simulink model "UDP_INTEGRATION_TEST_01"  (Simulink 8.1)
settings: Solver=ode4  StartTime=0.0  StopTime=inf  FixedStep=Ts  MaxStep=1e-3  RelTol=1e-3
PostLoadFcn:
  | INTEGRATION_TEST_01_init;
InitFcn:
  | INTEGRATION_TEST_01_init;
values from neighbouring files (symbols this model uses):
  Ts = 100E-6    (= 0.0001)    [INTEGRATION_TEST_01_init.m]
undefined symbols (not defined in the file or in its folder): cable_spec, fdesignblkfcn, gcbh, Left, relay_par, type, V
libraries: powerlib_extras x14, rtio_opalrt_common x13, rtlab x8, cables_lib x6, breaker_lib x4, simulink_extras x4, simulink x4, Load_lib x3, rtio_generic_modbus x3, powerlib x2, ssn_lib x2, transformer_lib x2
(part 2 of 2)

== system UDP_INTEGRATION_TEST_01/SS_Relays_and_Woodward/HWCtrl/SEL751_DigitalAnalog_IO_OpBlocks ==
  note: This connector also services Genset #2 and  is
      | shared with Genset #1.  Use RJ45 connectors to
      |  intercept Genset #2 I/O (not used in this Device
      | Integration Test) and use for SEL-751
  note: Remove existing connections to Slot 3 I/O, if any
      | ans replace with connections shown below, or use
      | corresponding RJ45 connectors.  (Existing I/O, if any not
      |  used for this Device Integration Test)
  note: When the system uses the simulated
      | Secondary Controller the digital I/O
      | should be disabled.
  note: Copyright (c) 2016 Massachusetts Institute of Technology
      | Permission is hereby granted, free of charge, to any person obtaining a copy of this software and associated documentation files (the "Software"), to deal
      | in the Software without restriction, including without limitation the rights to use, copy, modify, merge, publish, distribute, sublicense, and/or sell copies of the
      | Software, and to permit persons to whom the Software is furnished to do so, subject to the following conditions:
      |
      | THE SOFTWARE IS PROVIDED "AS IS", WITHOUT WARRANTY OF ANY KIND, EXPRESS OR IMPLIED, INCLUDING BUT NOT LIMITED TO THE
      | WARRANTIES OF MERCHANTABILITY, FITNESS FOR A PARTICULAR PURPOSE AND NONINFRINGEMENT. IN NO EVENT SHALL THE AUTHORS
      | OR COPYRIGHT HOLDERS BE LIABLE FOR ANY CLAIM, DAMAGES OR OTHER LIABILITY, WHETHER IN AN ACTION OF CONTRACT, TORT OR
      | OTHERWISE, ARISING FROM, OUT OF OR IN CONNECTION WITH THE SOFTWARE OR THE USE OR OTHER DEALINGS IN THE SOFTWARE
  SEL751-01_ScaledSignals : Inport
  AnalogOut2 to SEL-751 : rtio_opalrt_common/AnalogOut  CtrlName='OpCtrl'  portNb=4  FcnNos=Slot 2 Module A Subsection 2  size=16  maxcount=8  count=8  numchan=8  israngeinput=off  voltagerange=[ -5 ... 5 ]  slot=1  side=0  mismatch=0  slotside=Slot_2_Module_A
      settings: AttributesFormatString=%<CtrlName>
  Bus Creator4 : BusCreator  Inputs=2
  Bus Selector4 : BusSelector  OutputSignals=To DigitalOut_to_SEL-751,To AnalogOut_to_SEL-751
  Data Type Conversion{,1..3} (4 alike) : DataTypeConversion
  Demux6 : Demux  Outputs=8
  DigitalIn from SEL-751 : rtio_opalrt_common/DigitalIn  CtrlName='OpCtrl'  portNb=6  FcnNos=Slot 3 Module A Subsection 2  size=1  maxcount=8  count=8  sampleTime=Ts  numchan=8
      settings: AttributesFormatString=%<CtrlName>
  DigitalOut to SEL-751 : rtio_opalrt_common/DigitalOut  CtrlName='OpCtrl'  portNb=6  FcnNos=Slot 3 Module B Subsection 2  size=1  maxcount=8  count=8  numchan=8
      settings: AttributesFormatString=%<CtrlName>
  S-R Flip-Flop : simulink_extras/Flip Flops/S-R Flip-Flop  initial_condition=1
  Terminator : Terminator
  Terminator1 : Terminator
  Terminator2 : Terminator
  SEL751-01_LogicTrip : Outport
  wires:
  DigitalOut to SEL-751/1 -> Terminator1/1
  AnalogOut2 to SEL-751/1 -> Terminator/1
  Demux6/2 -> Data Type Conversion1/1  "OUT102 Brkr reset"
  Demux6/1 -> Data Type Conversion/1  "OUT103 Brkr trip"
  Data Type Conversion3/1 -> Bus Creator4/2  "Logic_reset"
  Data Type Conversion/1 -> S-R Flip-Flop/1
  Bus Selector4/2 -> AnalogOut2 to SEL-751/1  "<To AnalogOut_to_SEL-751>"
  Bus Selector4/1 -> DigitalOut to SEL-751/1  "<To DigitalOut_to_SEL-751>"
  DigitalIn from SEL-751/2 -> Terminator2/1
  SEL751-01_ScaledSignals/1 -> Bus Selector4/1
  DigitalIn from SEL-751/1 -> Demux6/1
  Data Type Conversion1/1 -> S-R Flip-Flop/2
  Data Type Conversion2/1 -> Bus Creator4/1  "Logic_trip"
  Bus Creator4/1 -> SEL751-01_LogicTrip/1
  S-R Flip-Flop/1 -> Data Type Conversion2/1  "Logic_trip"
  S-R Flip-Flop/2 -> Data Type Conversion3/1  "Logic_reset"

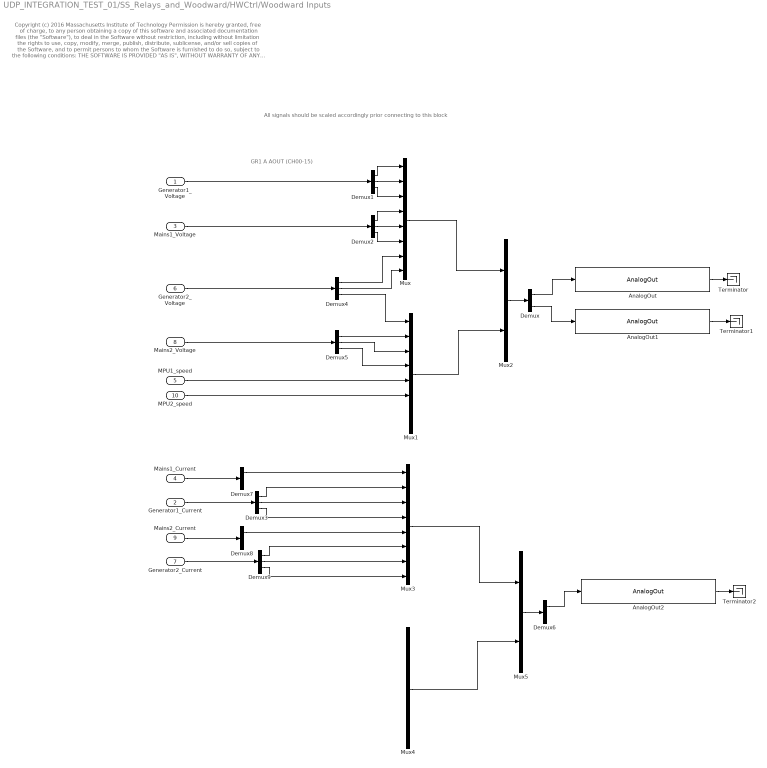
== system UDP_INTEGRATION_TEST_01/SS_Relays_and_Woodward/HWCtrl/Woodward Inputs ==
  note: All signals should be scaled accordingly prior connecting to this block
  note: GR1 A AOUT (CH00-15)
  note: Copyright (c) 2016 Massachusetts Institute of Technology
      | Permission is hereby granted, free of charge, to any person obtaining a copy of this software and associated documentation files (the "Software"), to deal
      | in the Software without restriction, including without limitation the rights to use, copy, modify, merge, publish, distribute, sublicense, and/or sell copies of the
      | Software, and to permit persons to whom the Software is furnished to do so, subject to the following conditions:
      |
      | THE SOFTWARE IS PROVIDED "AS IS", WITHOUT WARRANTY OF ANY KIND, EXPRESS OR IMPLIED, INCLUDING BUT NOT LIMITED TO THE
      | WARRANTIES OF MERCHANTABILITY, FITNESS FOR A PARTICULAR PURPOSE AND NONINFRINGEMENT. IN NO EVENT SHALL THE AUTHORS
      | OR COPYRIGHT HOLDERS BE LIABLE FOR ANY CLAIM, DAMAGES OR OTHER LIABILITY, WHETHER IN AN ACTION OF CONTRACT, TORT OR
      | OTHERWISE, ARISING FROM, OUT OF OR IN CONNECTION WITH THE SOFTWARE OR THE USE OR OTHER DEALINGS IN THE SOFTWARE
  Generator1_Voltage : Inport
  Generator1_Current : Inport  Port=2
  Mains1_Voltage : Inport  Port=3
  Mains1_Current : Inport  Port=4
  MPU1_speed : Inport  Port=5
  Generator2_Voltage : Inport  Port=6
  Generator2_Current : Inport  Port=7
  Mains2_Voltage : Inport  Port=8
  Mains2_Current : Inport  Port=9
  MPU2_speed : Inport  Port=10
  AnalogOut : rtio_opalrt_common/AnalogOut  CtrlName='OpCtrl'  portNb=1  FcnNos=Slot 1 Module A Subsection 1  size=16  maxcount=8  count=8  numchan=8  israngeinput=off  voltagerange=[-16 ... 16]  slot=0  side=0  mismatch=0  slotside=Slot_1_Module_A
      settings: AttributesFormatString=%<CtrlName>
  AnalogOut1 : rtio_opalrt_common/AnalogOut  CtrlName='OpCtrl'  portNb=2  FcnNos=Slot 1 Module A Subsection 2  size=16  maxcount=8  count=8  numchan=8  israngeinput=off  voltagerange=[-16 ... 16]  slot=0  side=0  mismatch=0  slotside=Slot_1_Module_A
      settings: AttributesFormatString=%<CtrlName>
  AnalogOut2 : rtio_opalrt_common/AnalogOut  CtrlName='OpCtrl'  portNb=3  FcnNos=Slot 2 Module A Subsection 1  size=16  maxcount=8  count=8  numchan=8  israngeinput=off  voltagerange=[-16 ... 16]  slot=1  side=0  mismatch=0  slotside=Slot_2_Module_A
      settings: AttributesFormatString=%<CtrlName>
  Demux : Demux  Outputs=2
  Demux{1..5,7..9} (8 alike) : Demux  Outputs=3
  Demux6 : Demux  Outputs=2
  Mux{,1,3..4} (4 alike) : Mux  Inputs=8
  Mux2 : Mux  Inputs=2
  Mux5 : Mux  Inputs=2
  Terminator : Terminator
  Terminator1 : Terminator
  Terminator2 : Terminator
  wires:
  Demux9/3 -> Mux3/8
  Demux9/2 -> Mux3/7
  Demux9/1 -> Mux3/6
  Generator2_Current/1 -> Demux9/1
  Demux8/1 -> Mux3/5
  Mains2_Current/1 -> Demux8/1
  MPU2_speed/1 -> Mux1/6
  Generator2_Voltage/1 -> Demux4/1
  Mains2_Voltage/1 -> Demux5/1
  Demux7/1 -> Mux3/1
  Mains1_Current/1 -> Demux7/1
  Demux3/3 -> Mux3/4
  Demux3/2 -> Mux3/3
  Demux3/1 -> Mux3/2
  Generator1_Current/1 -> Demux3/1
  AnalogOut2/1 -> Terminator2/1
  Demux6/1 -> AnalogOut2/1
  Mux3/1 -> Mux5/1
  Mux4/1 -> Mux5/2
  Mux5/1 -> Demux6/1
  Demux5/3 -> Mux1/4
  Demux5/2 -> Mux1/3
  Demux5/1 -> Mux1/2
  Demux4/3 -> Mux1/1
  Demux4/2 -> Mux/8
  Demux4/1 -> Mux/7
  MPU1_speed/1 -> Mux1/5
  Demux2/3 -> Mux/6
  Demux2/2 -> Mux/5
  Demux2/1 -> Mux/4
  Demux1/3 -> Mux/3
  Demux1/2 -> Mux/2
  Demux1/1 -> Mux/1
  AnalogOut/1 -> Terminator/1
  AnalogOut1/1 -> Terminator1/1
  Demux/1 -> AnalogOut/1
  Demux/2 -> AnalogOut1/1
  Mux/1 -> Mux2/1
  Mux1/1 -> Mux2/2
  Mux2/1 -> Demux/1
  Generator1_Voltage/1 -> Demux1/1
  Mains1_Voltage/1 -> Demux2/1

== system UDP_INTEGRATION_TEST_01/SS_Relays_and_Woodward/HWCtrl/Woodward Outputs - NGCHP - Gen1 ==
  note: Copyright (c) 2016 Massachusetts Institute of Technology
      | Permission is hereby granted, free of charge, to any person obtaining a copy of this software and associated documentation files (the "Software"), to deal
      | in the Software without restriction, including without limitation the rights to use, copy, modify, merge, publish, distribute, sublicense, and/or sell copies of the
      | Software, and to permit persons to whom the Software is furnished to do so, subject to the following conditions:
      |
      | THE SOFTWARE IS PROVIDED "AS IS", WITHOUT WARRANTY OF ANY KIND, EXPRESS OR IMPLIED, INCLUDING BUT NOT LIMITED TO THE
      | WARRANTIES OF MERCHANTABILITY, FITNESS FOR A PARTICULAR PURPOSE AND NONINFRINGEMENT. IN NO EVENT SHALL THE AUTHORS
      | OR COPYRIGHT HOLDERS BE LIABLE FOR ANY CLAIM, DAMAGES OR OTHER LIABILITY, WHETHER IN AN ACTION OF CONTRACT, TORT OR
      | OTHERWISE, ARISING FROM, OUT OF OR IN CONNECTION WITH THE SOFTWARE OR THE USE OR OTHER DEALINGS IN THE SOFTWARE
  Gen1 MCB Status : Inport
  WoodwardBias : Inport  Port=2
  Bus Creator1 : BusCreator  Inputs=1
  DIO - Gr3 : Subsystem
  DIO - Woodward : Subsystem
  DOUT type config : Subsystem
  Woodward Primary Inputs - Gen1 : Subsystem
  Digital Inputs : Outport
  Gen1 Gov and AVR : Outport  Port=2
  Gen1 Fuel Enable : Outport  Port=3
  Gen1 GCB : Outport  Port=4
  Gen1 MCB : Outport  Port=5
  wires:
  Gen1 MCB Status/1 -> DIO - Woodward/2(Gen1 MCB Status)
  DIO - Woodward/1(Gen1 Fuel Enable) -> Gen1 Fuel Enable/1
  DIO - Woodward/3(Gen1 MCB) -> Gen1 MCB/1
  DIO - Woodward/2(Gen1 GCB) -> Gen1 GCB/1
  WoodwardBias/1 -> Woodward Primary Inputs - Gen1/1(WoodwardBias)
  Woodward Primary Inputs - Gen1/1(Gen1 Gov and AVR) -> Gen1 Gov and AVR/1
  Bus Creator1/1 -> Digital Inputs/1
  DIO - Gr3/1(DIn) -> Bus Creator1/1, DIO - Woodward/1(Din_Wood)  "DIN"
  DIO - Woodward/4(DIn1) -> DIO - Gr3/1(Dout)

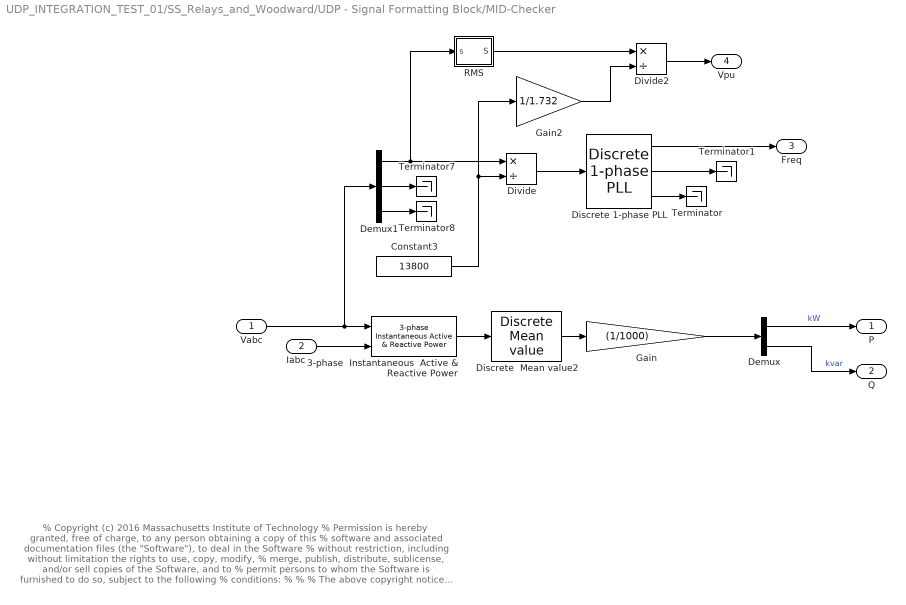
== system UDP_INTEGRATION_TEST_01/SS_Relays_and_Woodward/UDP - Signal Formatting Block/MID-Checker ==
  note: % Copyright (c) 2016 Massachusetts Institute of Technology
      | % Permission is hereby granted, free of charge, to any person obtaining a copy of this
      | % software and associated documentation files (the "Software"), to deal in the Software
      | % without restriction, including without limitation the rights to use, copy, modify,
      | % merge, publish, distribute, sublicense, and/or sell copies of the Software, and to
      | % permit persons to whom the Software is furnished to do so, subject to the following
      | % conditions:
      | %
      | %
      | % The above copyright notice and this permission notice shall be included in
      | % all copies or substantial portions of the Software.
      | %
      | % THE SOFTWARE IS PROVIDED "AS IS", WITHOUT WARRANTY OF ANY KIND, EXPRESS OR IMPLIED,
      | % INCLUDING BUT NOT LIMITED TO THE WARRANTIES OF MERCHANTABILITY, FITNESS FOR A
      | % PARTICULAR PURPOSE AND NONINFRINGEMENT. IN NO EVENT SHALL THE AUTHORS OR COPYRIGHT
      | % HOLDERS BE LIABLE FOR ANY CLAIM, DAMAGES OR OTHER LIABILITY, WHETHER IN AN ACTION
      | % OF CONTRACT, TORT OR OTHERWISE, ARISING FROM, OUT OF OR IN CONNECTION WITH THE
      | % SOFTWARE OR THE USE OR OTHER DEALINGS IN THE SOFTWARE.
      | %
      | %
      | %%
  Vabc : Inport
  Iabc : Inport  Port=2
  3-phase  Instantaneous  Active & Reactive Power : powerlib_extras/Measurements/3-phase  Instantaneous  Active & Reactive Power
  Constant3 : Constant  Value=13800
  Demux : Demux  Outputs=2
  Demux1 : Demux  Outputs=3
  Discrete 1-phase PLL : powerlib_extras/Discrete  Control Blocks/Discrete 1-phase PLL  Fmin=45  Par_Init=[0 60]  ParK=[ 180 3200 1]  Ts=Ts  AGC=on
  Discrete  Mean value2 : powerlib_extras/Discrete Measurements/Discrete  Mean value  Freq=60  Vinit=0  Ts=Ts
  Divide : Product  Inputs=*/
  Divide2 : Product  Inputs=*/
  Gain : Gain  Gain=(1/1000)
  Gain2 : Gain  Gain=1/1.732
  RMS : Subsystem
  Terminator{,1,7..8} (4 alike) : Terminator
  P : Outport
  Q : Outport  Port=2
  Freq : Outport  Port=3
  Vpu : Outport  Port=4
  wires:
  Demux/2 -> Q/1  "kvar"
  Demux/1 -> P/1  "kW"
  Iabc/1 -> 3-phase  Instantaneous  Active & Reactive Power/2
  Discrete  Mean value2/1 -> Gain/1
  3-phase  Instantaneous  Active & Reactive Power/1 -> Discrete  Mean value2/1
  Gain/1 -> Demux/1
  Discrete 1-phase PLL/1 -> Freq/1
  Discrete 1-phase PLL/3 -> Terminator/1
  Divide/1 -> Discrete 1-phase PLL/1
  Discrete 1-phase PLL/2 -> Terminator1/1
  Demux1/1 -> RMS/1(s), Divide/1
  Demux1/2 -> Terminator7/1
  Demux1/3 -> Terminator8/1
  Vabc/1 -> 3-phase  Instantaneous  Active & Reactive Power/1, Demux1/1
  Constant3/1 -> Divide/2, Gain2/1
  Gain2/1 -> Divide2/2
  RMS/1(S) -> Divide2/1
  Divide2/1 -> Vpu/1

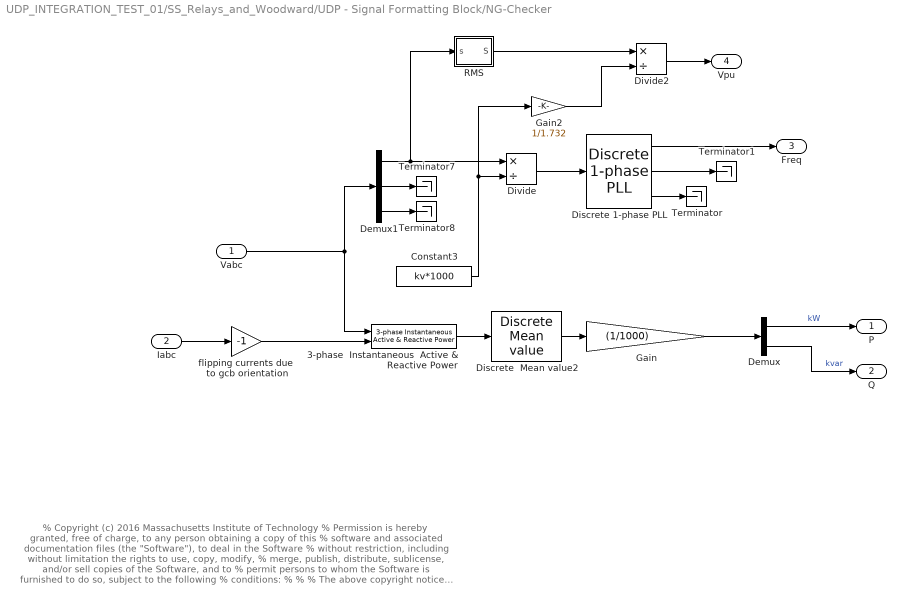
== system UDP_INTEGRATION_TEST_01/SS_Relays_and_Woodward/UDP - Signal Formatting Block/NG-Checker ==
  note: % Copyright (c) 2016 Massachusetts Institute of Technology
      | % Permission is hereby granted, free of charge, to any person obtaining a copy of this
      | % software and associated documentation files (the "Software"), to deal in the Software
      | % without restriction, including without limitation the rights to use, copy, modify,
      | % merge, publish, distribute, sublicense, and/or sell copies of the Software, and to
      | % permit persons to whom the Software is furnished to do so, subject to the following
      | % conditions:
      | %
      | %
      | % The above copyright notice and this permission notice shall be included in
      | % all copies or substantial portions of the Software.
      | %
      | % THE SOFTWARE IS PROVIDED "AS IS", WITHOUT WARRANTY OF ANY KIND, EXPRESS OR IMPLIED,
      | % INCLUDING BUT NOT LIMITED TO THE WARRANTIES OF MERCHANTABILITY, FITNESS FOR A
      | % PARTICULAR PURPOSE AND NONINFRINGEMENT. IN NO EVENT SHALL THE AUTHORS OR COPYRIGHT
      | % HOLDERS BE LIABLE FOR ANY CLAIM, DAMAGES OR OTHER LIABILITY, WHETHER IN AN ACTION
      | % OF CONTRACT, TORT OR OTHERWISE, ARISING FROM, OUT OF OR IN CONNECTION WITH THE
      | % SOFTWARE OR THE USE OR OTHER DEALINGS IN THE SOFTWARE.
      | %
      | %
      | %%
  Vabc : Inport
  Iabc : Inport  Port=2
  3-phase  Instantaneous  Active & Reactive Power : powerlib_extras/Measurements/3-phase  Instantaneous  Active & Reactive Power
  Constant3 : Constant  Value=kv*1000
  Demux : Demux  Outputs=2
  Demux1 : Demux  Outputs=3
  Discrete 1-phase PLL : powerlib_extras/Discrete  Control Blocks/Discrete 1-phase PLL  Fmin=45  Par_Init=[0 60]  ParK=[ 180 3200 1]  Ts=Ts  AGC=on
  Discrete  Mean value2 : powerlib_extras/Discrete Measurements/Discrete  Mean value  Freq=60  Vinit=0  Ts=Ts
  Divide : Product  Inputs=*/
  Divide2 : Product  Inputs=*/
  Gain : Gain  Gain=(1/1000)
  Gain2 : Gain  Gain=1/1.732
  RMS : Subsystem
  Terminator{,1,7..8} (4 alike) : Terminator
  flipping currents due  to gcb orientation : Gain  Gain=-1
  P : Outport
  Q : Outport  Port=2
  Freq : Outport  Port=3
  Vpu : Outport  Port=4
  wires:
  Demux/2 -> Q/1  "kvar"
  Demux/1 -> P/1  "kW"
  Iabc/1 -> flipping currents due  to gcb orientation/1
  Discrete  Mean value2/1 -> Gain/1
  3-phase  Instantaneous  Active & Reactive Power/1 -> Discrete  Mean value2/1
  Gain/1 -> Demux/1
  Discrete 1-phase PLL/1 -> Freq/1
  Discrete 1-phase PLL/3 -> Terminator/1
  Divide/1 -> Discrete 1-phase PLL/1
  Discrete 1-phase PLL/2 -> Terminator1/1
  Demux1/1 -> RMS/1(s), Divide/1
  Demux1/2 -> Terminator7/1
  Demux1/3 -> Terminator8/1
  Vabc/1 -> 3-phase  Instantaneous  Active & Reactive Power/1, Demux1/1
  Constant3/1 -> Divide/2, Gain2/1
  Gain2/1 -> Divide2/2
  RMS/1(S) -> Divide2/1
  Divide2/1 -> Vpu/1
  flipping currents due  to gcb orientation/1 -> 3-phase  Instantaneous  Active & Reactive Power/2

== system UDP_INTEGRATION_TEST_01/SS_Relays_and_Woodward/UDP - Signal Formatting Block/RMS ==
  s : Inport
  Discrete  Mean value6 : powerlib_extras/Discrete Measurements/Discrete  Mean value  Freq=60  Vinit=0  Ts=Ts
  Product3 : Product  RndMeth=Zero
  Signed Sqrt : Sqrt  SaturateOnIntegerOverflow=on
  S : Outport
  wires:
  Signed Sqrt/1 -> S/1
  Discrete  Mean value6/1 -> Signed Sqrt/1
  Product3/1 -> Discrete  Mean value6/1
  s/1 -> Product3/2, Product3/1

== system UDP_INTEGRATION_TEST_01/SS_Relays_and_Woodward/UDP - Signal Formatting Block/set of 1ph PLLs ==
  V_bus : Inport
  V_line : Inport  Port=2
  VRMSLL : Inport  Port=3
  Discrete 1-phase PLL : powerlib_extras/Discrete  Control Blocks/Discrete 1-phase PLL  Fmin=45  Par_Init=[0 60]  ParK=[ 180 3200 1]  Ts=Ts  AGC=on
  Discrete 1-phase PLL1 : powerlib_extras/Discrete  Control Blocks/Discrete 1-phase PLL  Fmin=45  Par_Init=[0 60]  ParK=[ 180 3200 1]  Ts=Ts  AGC=on
  Divide : Product  Inputs=*/
  Divide1 : Product  Inputs=*/
  Terminator : Terminator
  Terminator1 : Terminator
  f_bus : Outport
  f_line : Outport  Port=2
  wt_bus : Outport  Port=3
  wt_line : Outport  Port=4
  wires:
  V_bus/1 -> Divide1/1
  Divide1/1 -> Discrete 1-phase PLL1/1
  V_line/1 -> Divide/1
  Divide/1 -> Discrete 1-phase PLL/1
  VRMSLL/1 -> Divide1/2, Divide/2
  Discrete 1-phase PLL1/1 -> f_bus/1
  Discrete 1-phase PLL1/2 -> wt_bus/1
  Discrete 1-phase PLL/1 -> f_line/1
  Discrete 1-phase PLL/2 -> wt_line/1
  Discrete 1-phase PLL/3 -> Terminator/1
  Discrete 1-phase PLL1/3 -> Terminator1/1

== system UDP_INTEGRATION_TEST_01/SS_Relays_and_Woodward/HWCtrl/Woodward Outputs - NGCHP - Gen1/DIO - Gr3 ==
  Dout : Inport
  Bus Creator : BusCreator  Inputs=1
  Bus Selector : BusSelector  OutputSignals=DI_CH00-07  OutputAsBus=on
  Conditioning : Subsystem
  DigitalIn : rtio_opalrt_common/DigitalIn  CtrlName='OpCtrl'  portNb=5  FcnNos=Slot 3 Module A Subsection 1  size=1  maxcount=8  count=8  sampleTime=0  numchan=8
      settings: AttributesFormatString=%<CtrlName>
  DigitalOut : rtio_opalrt_common/DigitalOut  CtrlName='OpCtrl'  portNb=5  FcnNos=Slot 3 Module B Subsection 1  size=1  maxcount=8  count=8  numchan=8
      settings: AttributesFormatString=%<CtrlName>
  Terminator3 : Terminator
  Terminator5 : Terminator
  DIn : Outport
  wires:
  Conditioning/1(Out1) -> Bus Creator/1
  Bus Creator/1 -> DIn/1
  DigitalIn/1 -> Conditioning/1(In1)  "DI_CH00-07"
  DigitalIn/2 -> Terminator5/1
  Bus Selector/1 -> DigitalOut/1
  Dout/1 -> Bus Selector/1
  DigitalOut/1 -> Terminator3/1

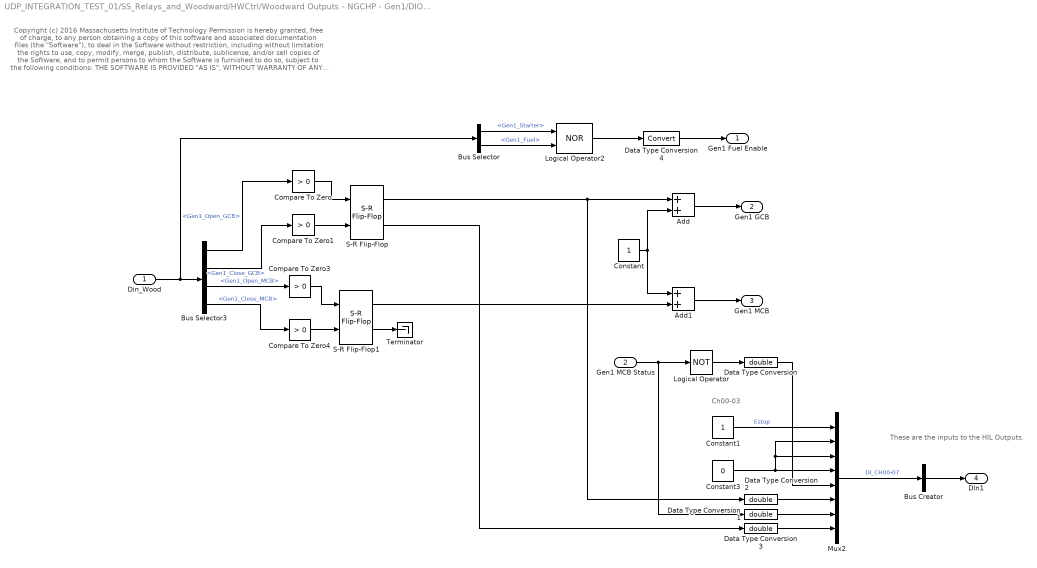
== system UDP_INTEGRATION_TEST_01/SS_Relays_and_Woodward/HWCtrl/Woodward Outputs - NGCHP - Gen1/DIO - Woodward ==
  note: Copyright (c) 2016 Massachusetts Institute of Technology
      | Permission is hereby granted, free of charge, to any person obtaining a copy of this software and associated documentation files (the "Software"), to deal
      | in the Software without restriction, including without limitation the rights to use, copy, modify, merge, publish, distribute, sublicense, and/or sell copies of the
      | Software, and to permit persons to whom the Software is furnished to do so, subject to the following conditions:
      |
      | THE SOFTWARE IS PROVIDED "AS IS", WITHOUT WARRANTY OF ANY KIND, EXPRESS OR IMPLIED, INCLUDING BUT NOT LIMITED TO THE
      | WARRANTIES OF MERCHANTABILITY, FITNESS FOR A PARTICULAR PURPOSE AND NONINFRINGEMENT. IN NO EVENT SHALL THE AUTHORS
      | OR COPYRIGHT HOLDERS BE LIABLE FOR ANY CLAIM, DAMAGES OR OTHER LIABILITY, WHETHER IN AN ACTION OF CONTRACT, TORT OR
      | OTHERWISE, ARISING FROM, OUT OF OR IN CONNECTION WITH THE SOFTWARE OR THE USE OR OTHER DEALINGS IN THE SOFTWARE
  note: Ch00-03
  note: These are the inputs to
      | the HIL Outputs.
  Din_Wood : Inport
  Gen1 MCB Status : Inport  Port=2
  Add : Sum
  Add1 : Sum
  Bus Creator : BusCreator  Inputs=1
  Bus Selector : BusSelector  OutputSignals=DI_CH00-07.Gen1_Starter,DI_CH00-07.Gen1_Fuel
  Bus Selector3 : BusSelector  OutputSignals=DI_CH00-07.Gen1_Open_GCB,DI_CH00-07.Gen1_Close_GCB,DI_CH00-07.Gen1_Open_MCB,DI_CH00-07.Gen1_Close_MCB
  Compare To Zero{,1,3..4} (4 alike) : simulink/Logic and Bit Operations/Compare To Zero  relop=>  OutDataTypeStr=boolean
  Constant : Constant
  Constant1 : Constant
  Constant3 : Constant  Value=0
  Data Type Conversion{,1..3} (4 alike) : DataTypeConversion  OutDataTypeStr=double
  Data Type Conversion4 : DataTypeConversion
  Logical Operator : Logic  Operator=NOT  AllPortsSameDT=off  OutDataTypeStr=boolean
  Logical Operator2 : Logic  Operator=NOR  AllPortsSameDT=off  OutDataTypeStr=boolean
  Mux2 : Mux  Inputs=8
  S-R Flip-Flop : simulink_extras/Flip Flops/S-R Flip-Flop  initial_condition=1
  S-R Flip-Flop1 : simulink_extras/Flip Flops/S-R Flip-Flop  initial_condition=1
  Terminator : Terminator
  Gen1 Fuel Enable : Outport
  Gen1 GCB : Outport  Port=2
  Gen1 MCB : Outport  Port=3
  DIn1 : Outport  Port=4
  wires:
  S-R Flip-Flop1/2 -> Terminator/1
  Data Type Conversion2/1 -> Mux2/6
  Data Type Conversion1/1 -> Mux2/7
  Data Type Conversion3/1 -> Mux2/8
  Mux2/1 -> Bus Creator/1  "DI_CH00-07"
  Constant3/1 -> Mux2/2, Mux2/3, Mux2/4
  Logical Operator2/1 -> Data Type Conversion4/1
  Logical Operator/1 -> Data Type Conversion/1
  Data Type Conversion/1 -> Mux2/5
  S-R Flip-Flop/2 -> Data Type Conversion3/1
  Gen1 MCB Status/1 -> Logical Operator/1, Data Type Conversion1/1
  Bus Selector3/3 -> Compare To Zero3/1  "<Gen1_Open_MCB>"
  Bus Selector/2 -> Logical Operator2/2  "<Gen1_Fuel>"
  Bus Selector/1 -> Logical Operator2/1  "<Gen1_Starter>"
  Constant/1 -> Add1/1, Add/2
  Add1/1 -> Gen1 MCB/1
  Add/1 -> Gen1 GCB/1
  S-R Flip-Flop1/1 -> Add1/2
  Compare To Zero3/1 -> S-R Flip-Flop1/1
  Compare To Zero4/1 -> S-R Flip-Flop1/2
  Bus Selector3/4 -> Compare To Zero4/1  "<Gen1_Close_MCB>"
  Compare To Zero1/1 -> S-R Flip-Flop/2
  Compare To Zero/1 -> S-R Flip-Flop/1
  S-R Flip-Flop/1 -> Data Type Conversion2/1, Add/1
  Bus Creator/1 -> DIn1/1
  Din_Wood/1 -> Bus Selector/1, Bus Selector3/1
  Bus Selector3/1 -> Compare To Zero/1  "<Gen1_Open_GCB>"
  Bus Selector3/2 -> Compare To Zero1/1  "<Gen1_Close_GCB>"
  Data Type Conversion4/1 -> Gen1 Fuel Enable/1
  Constant1/1 -> Mux2/1  "Estop"

== system UDP_INTEGRATION_TEST_01/SS_Relays_and_Woodward/HWCtrl/Woodward Outputs - NGCHP - Gen1/DOUT type config ==
  note: The Constants are used to select Digital Output type:
      | - 0: Time-Stamped Digital Output
      | - 1: Pulse-Width Modulated DIgital Output
  DataIn Send : rtio_opalrt_common/DataIn Send  CtrlName='OpCtrl'  FcnNos=11  width=1  portType=double  checkVersion=off  expectedId=0  expectedVersion=0  opComp=>=
      settings: AttributesFormatString=%<CtrlName>
  DataIn Send1 : rtio_opalrt_common/DataIn Send  CtrlName='OpCtrl'  FcnNos=12  width=1  portType=double  checkVersion=off  expectedId=0  expectedVersion=0  opComp=>=
      settings: AttributesFormatString=%<CtrlName>
  Subsection 3 DOUT type : Constant
  Subsection 4 DOUT type : Constant
  Terminator1 : Terminator
  Terminator2 : Terminator
  wires:
  DataIn Send/1 -> Terminator2/1
  DataIn Send1/1 -> Terminator1/1
  Subsection 4 DOUT type/1 -> DataIn Send1/1
  Subsection 3 DOUT type/1 -> DataIn Send/1

== system UDP_INTEGRATION_TEST_01/SS_Relays_and_Woodward/HWCtrl/Woodward Outputs - NGCHP - Gen1/Woodward Primary Inputs - Gen1 ==
  note: Copyright (c) 2016 Massachusetts Institute of Technology
      | Permission is hereby granted, free of charge, to any person obtaining a copy of this software and associated documentation files (the "Software"), to deal
      | in the Software without restriction, including without limitation the rights to use, copy, modify, merge, publish, distribute, sublicense, and/or sell copies of the
      | Software, and to permit persons to whom the Software is furnished to do so, subject to the following conditions:
      |
      | THE SOFTWARE IS PROVIDED "AS IS", WITHOUT WARRANTY OF ANY KIND, EXPRESS OR IMPLIED, INCLUDING BUT NOT LIMITED TO THE
      | WARRANTIES OF MERCHANTABILITY, FITNESS FOR A PARTICULAR PURPOSE AND NONINFRINGEMENT. IN NO EVENT SHALL THE AUTHORS
      | OR COPYRIGHT HOLDERS BE LIABLE FOR ANY CLAIM, DAMAGES OR OTHER LIABILITY, WHETHER IN AN ACTION OF CONTRACT, TORT OR
      | OTHERWISE, ARISING FROM, OUT OF OR IN CONNECTION WITH THE SOFTWARE OR THE USE OR OTHER DEALINGS IN THE SOFTWARE
  note: NG-CHP -> Gen1
  WoodwardBias : Inport
  Bus Creator : BusCreator
  Bus Selector5 : BusSelector  OutputSignals=gen1_GOV_bias,gen1_AVR_bias
  Constant3 : Constant  Value=0
  Constant4 : Constant  Value=0
  Divide : Product  Inputs=*/
  Divide1 : Product  Inputs=*/
  Gen1 Ref AVR : Constant  Value=1.00
  Gen1 Ref GOV : Constant  Value=1.00
  Lowpass Filter : Subsystem  DialogController=fdesignblkfcn  DialogControllerArgs=DataTag2  InitFcn=fdesignblkfcn(gcbh, {'InitFcn'});  mask(Lowpass Filter){}
      mask help: Design a lowpass filter
      settings: CopyFcn=fdesignblkfcn(gcbh, {'CopyFcn'});
      mask Help: helpview(mapfilelocation('dsp'), 'dsplowpassfilter');
      mask Display: disp('Lowpass')
  Lowpass Filter1 : Subsystem  DialogController=fdesignblkfcn  DialogControllerArgs=DataTag4  InitFcn=fdesignblkfcn(gcbh, {'InitFcn'});  mask(Lowpass Filter){}
      mask help: Design a lowpass filter
      settings: CopyFcn=fdesignblkfcn(gcbh, {'CopyFcn'});
      mask Help: helpview(mapfilelocation('dsp'), 'dsplowpassfilter');
      mask Display: disp('Lowpass')
  ScalingBias : Constant  Value=20
  SimulatedBiasValues : Constant  Value=0
  Sum : Sum  Inputs=|+-
  Sum1 : Sum  Inputs=|+-
  Switch : Switch  Threshold=0.5
  Switch1 : Switch  Threshold=0.5
  bias_enable_for_woodward_ctrl : Constant
  Gen1 Gov and AVR : Outport
  wires:
  Bus Selector5/2 -> Divide1/1  "<gen1_AVR_bias>"
  Bus Selector5/1 -> Divide/1  "<gen1_GOV_bias>"
  WoodwardBias/1 -> Bus Selector5/1
  Bus Creator/1 -> Gen1 Gov and AVR/1
  Gen1 Ref GOV/1 -> Bus Creator/1  "Gen1 Ref GOV"
  Gen1 Ref AVR/1 -> Bus Creator/2  "Gen1 Ref AVR"
  Lowpass Filter1/1(Out) -> Switch1/1
  Lowpass Filter/1(Out) -> Switch/1
  bias_enable_for_woodward_ctrl/1 -> Switch/2, Switch1/2
  SimulatedBiasValues/1 -> Switch1/3, Switch/3
  Sum1/1 -> Lowpass Filter1/1(In)
  Switch1/1 -> Bus Creator/4  "Gen1 AVR"
  Switch/1 -> Bus Creator/3  "Gen1 Gov"
  Sum/1 -> Lowpass Filter/1(In)
  Constant4/1 -> Sum1/2
  Constant3/1 -> Sum/2
  Divide1/1 -> Sum1/1
  Divide/1 -> Sum/1
  ScalingBias/1 -> Divide1/2, Divide/2

== system UDP_INTEGRATION_TEST_01/SS_Relays_and_Woodward/UDP - Signal Formatting Block/MID-Checker/RMS ==
  s : Inport
  Discrete  Mean value6 : powerlib_extras/Discrete Measurements/Discrete  Mean value  Freq=60  Vinit=0  Ts=Ts
  Product3 : Product  RndMeth=Zero
  Signed Sqrt : Sqrt  SaturateOnIntegerOverflow=on
  S : Outport
  wires:
  s/1 -> Product3/1, Product3/2
  Product3/1 -> Discrete  Mean value6/1
  Discrete  Mean value6/1 -> Signed Sqrt/1
  Signed Sqrt/1 -> S/1

== system UDP_INTEGRATION_TEST_01/SS_Relays_and_Woodward/UDP - Signal Formatting Block/NG-Checker/RMS ==
  s : Inport
  Discrete  Mean value6 : powerlib_extras/Discrete Measurements/Discrete  Mean value  Freq=60  Vinit=0  Ts=Ts
  Product3 : Product  RndMeth=Zero
  Signed Sqrt : Sqrt  SaturateOnIntegerOverflow=on
  S : Outport
  wires:
  s/1 -> Product3/1, Product3/2
  Product3/1 -> Discrete  Mean value6/1
  Discrete  Mean value6/1 -> Signed Sqrt/1
  Signed Sqrt/1 -> S/1

== system UDP_INTEGRATION_TEST_01/SS_Relays_and_Woodward/HWCtrl/Woodward Outputs - NGCHP - Gen1/DIO - Gr3/Conditioning ==
  In1 : Inport
  Bus Creator : BusCreator  Inputs=8
  Demux : Demux  Outputs=8
  Out1 : Outport
  wires:
  In1/1 -> Demux/1
  Bus Creator/1 -> Out1/1  "DI_CH00-07"
  Demux/8 -> Bus Creator/8  "Gen1_Alarm_CF"
  Demux/7 -> Bus Creator/7  "Gen1_Alarm_AB"
  Demux/6 -> Bus Creator/6  "Gen1_Open_MCB"
  Demux/5 -> Bus Creator/5  "Gen1_Close_MCB"
  Demux/4 -> Bus Creator/4  "Gen1_Open_GCB"
  Demux/3 -> Bus Creator/3  "Gen1_Close_GCB"
  Demux/2 -> Bus Creator/2  "Gen1_Fuel"
  Demux/1 -> Bus Creator/1  "Gen1_Starter"

== system UDP_INTEGRATION_TEST_01/SS_Relays_and_Woodward/HWCtrl/Woodward Outputs - NGCHP - Gen1/Woodward Primary Inputs - Gen1/Lowpass Filter ==
  In : Inport
  Generated Filter Block : DiscreteFir  Tag=BlockMethodSubSystem  Coefficients=[0.0069552863617617106 0.014587901014631248 -0.0057896483056441538 -0.056861876528372622 -0.059476680260783142 0.076118200884714562 0.29579154768342669 0.40638624201187618 0.29579154768342669 0.076118200884714562 -0.059476680260783142 -0.056861876528372622 -0.0057896483056441538 0.014587901014631248 0.0069552863617617106]  InputProcessing=Columns as channels (frame based)
  Out : Outport
  wires:
  Generated Filter Block/1 -> Out/1
  In/1 -> Generated Filter Block/1

== system UDP_INTEGRATION_TEST_01/SS_Relays_and_Woodward/HWCtrl/Woodward Outputs - NGCHP - Gen1/Woodward Primary Inputs - Gen1/Lowpass Filter1 ==
  In : Inport
  Generated Filter Block : DiscreteFir  Tag=BlockMethodSubSystem  Coefficients=[0.0069552863617617106 0.014587901014631248 -0.0057896483056441538 -0.056861876528372622 -0.059476680260783142 0.076118200884714562 0.29579154768342669 0.40638624201187618 0.29579154768342669 0.076118200884714562 -0.059476680260783142 -0.056861876528372622 -0.0057896483056441538 0.014587901014631248 0.0069552863617617106]  InputProcessing=Columns as channels (frame based)
  Out : Outport
  wires:
  Generated Filter Block/1 -> Out/1
  In/1 -> Generated Filter Block/1
